simulink model "main_sim_mk14_final"  (R2024a)
settings: Solver=ode23t  StartTime=0.0  StopTime=0.2  MaxStep=5e-7  RelTol=1e-5
InitFcn:
  | sw_freq=40e3;
undefined symbols (not defined in the file or in its folder): Ion, Lithium
libraries: spsSeriesRLCBranchLib x10, spsMeanLib x8, spsCurrentMeasurementLib x6, spsMosfetLib x4, spsVoltageMeasurementLib x3, spsBatteryLib x2, simulink x2, spsControlledCurrentSourceLib x1, spsGroundLib x1, eeStairGenerator x1, spspowerguiLib x1
settings Model: SimulationMode=rapid-accelerator  Creator=adamo  LastModifiedBy=adamo
settings SolverCC: AllowMultiTaskInputOutput=on  ZeroCrossAlgorithm=Adaptive  SolverResetMethod=Robust  PositivePriorityOrder=on  DecoupledContinuousIntegration=on  MinimalZcImpactIntegration=on
settings OptimizationCC: ReuseModelBlockBuffer=off  SimCompilerOptimization=on
settings DebuggingCC: MaskedZcDiagnostic=none  IgnoredZcDiagnostic=none
settings HardwareCC: ProdHWDeviceType=AMD->x86-64 (Windows64)
settings ModelReferenceCC: EnableParallelModelReferenceBuilds=on  ParallelModelReferenceMATLABWorkerInit=Copy Base Workspace  ModelReferenceMinAlgLoopOccurrences=on
settings SFSimCC: SimHardwareAcceleration=native  SimTargetLang=C++
settings RTWCC: BuildConfiguration=Faster Runs  GPUComputeCapability=3.5
settings GRTTargetCC: OptimizeReductions=on

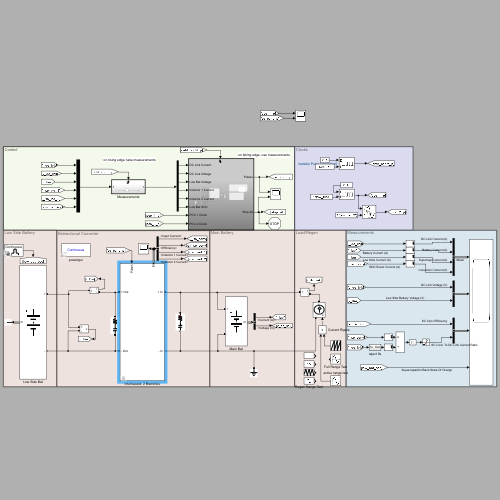
[thumbnail: Simulink's stored preview of the top-level diagram]
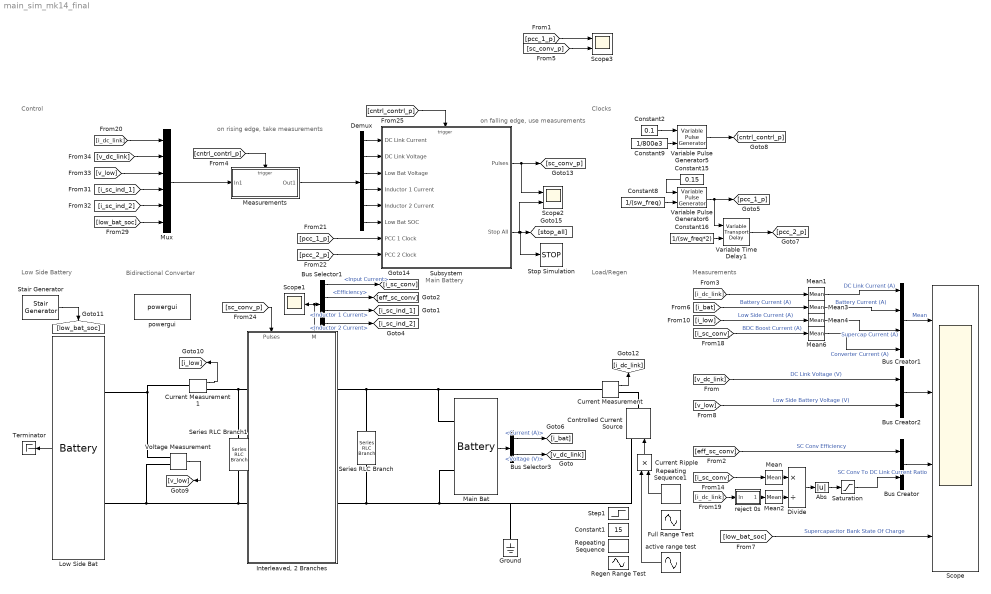
== system main_sim_mk14_final ==
  note: on falling edge, use measurements
  note: on rising edge, take measurements
  note: Clocks
  note: Control
  note: Measurements
  note: Bidirectional Converter
  note: Low Side Battery
  note: Main Battery
  note: Load/Regen
  Abs : Abs  SaturateOnIntegerOverflow=off
  Bus Creator : BusCreator  Inputs=2
  Bus Creator1 : BusCreator  Inputs=4
  Bus Creator2 : BusCreator  Inputs=2
  Bus Selector1 : BusSelector  OutputSignals=Input Current,Efficiency,Inductor 1 Current,Inductor 2 Current
  Bus Selector3 : BusSelector  OutputSignals=Current (A),Voltage (V)
  Constant1 : Constant  Value=15
  Constant15 : Constant  Value=0.15
  Constant16 : Constant  Value=1/(sw_freq*2)
  Constant2 : Constant  Value=0.1
  Constant8 : Constant  Value=1/(sw_freq)  VectorParams1D=off
  Constant9 : Constant  Value=1/800e3
  Controlled Current Source : spsControlledCurrentSourceLib/Controlled Current Source  Initialize=on  Source_Type=DC  Amplitude=0  Phase=0  Frequency=0  Measurements=None
  Current Measurement : spsCurrentMeasurementLib/Current Measurement  PhasorSimulation=off  OutputType=Complex  PSBequivalent=0
  Current Measurement1 : spsCurrentMeasurementLib/Current Measurement  PhasorSimulation=off  OutputType=Complex  PSBequivalent=0
  Current Ripple : Product
  Demux : Demux  Outputs=6
  Divide : Product  Inputs=*/
  Full Range Test : Sin  Amplitude=52  Frequency=314.1592/8  SampleTime=0
  Ground : spsGroundLib/Ground  LConnTagsString=a
  "Interleaved, 2 Branches" : Subsystem  mask{sw_freq_mean=sw_freq, ind_ind=200e-6, fet_res_on=10e-3, bd_d_for_volt=1.3}
      mask prompts: sw_freq_mean "Switching Frequency (Hz)"; ind_ind "Branch Inductor Inductance (H)"; fet_res_on "Drain-to-Source On-Resistance (Ohm)"; bd_d_for_volt "Body Diode Forward Voltage (V)"
      settings: PortSchema="{\"entries\":[{\"content\":{\"sides\":[{\"content\":{\"connectorIds\":[\"LConn1\",\"LConn2\"]},\"type\":\"ConnectorPlacement.EquallySpacedRectSide\",\"uuid\":\"57763a22-817d-4d04-a19a-6b084199baa7\"},{\"content\":{\"connectorIds\":[\"RConn1\",\"RConn2\"],\"side\":\"RIGHT\"},\"type\":\"ConnectorPlacement.EquallySpacedRectSide\",\"uuid\":\"e5f04f53-fac9-409a-ac58-f518a07f7aa1\"},{\"content\":{\"connectorIds\":[\"In1\",\"Out1\"],\"side\":\"TOP\"},\"type\":\"ConnectorPlacement.EquallySpacedRectSide\",\"uuid\":\"7683f119-33ed-4468-84c8-2aaaca937041\"}]},\"type\":\"ConnectorPlacement.EquallySpacedConnector\",\"uuid\":\"94c2a178-e796-4540-a87e-c79e0224e730\"}],\"packageUris\":[\"http://schema.mathworks.com/mf0/Connector/R2020b\"],\"version\":\"1.0\"}"
      mask DialogControl DescTextVar Prompt: %<MaskDescription>This block impements a Two Phase Interleaved Bidirectional DC-DC Buck/Boost Converter. Input is the left side (High Voltage Side). All MOSFETs share the same characteristics.
      mask DialogControl ParameterGroupVar Prompt: Circuit Parameters
      mask DialogControl Container3 Prompt: MOSFET Parameters
  Low Side Bat : spsBatteryLib/Battery  BatType=Lithium-Ion  ShowTempParam=off  ThermalPreset=no  ShowAgeParam=off  NomV=32  NomQ=30  SOC=75  Batt_Tr=30  PresetModel=on  MaxQ=30  MinV=24  FullV=37.2476  Dis_rate=13.0435  R=0.010667  Normal_OP=27.1304  expZone="[34.5723      1.47391]"  current=[6.5 13 32.5]  Units=Time  Tci=20  NomT=20  T2=-30  MaxQ2=4.8  FullV2=7.1  Normal_OP2=5.655  expZone2="[6.58           1]"  Rca=0.6  ti=2000  Dp=0  Neq0=0  Tsim=1e6  Ta1=25  Qeol=5.4*0.9  Reol=0.013333*1.2  Char_age=[2.3478, 3]  Dis_age=[2.3478, 10]  N1=1500  N2=10500  N3=1000  N4=1400  Ta2=45  N5=950
  Main Bat : spsBatteryLib/Battery  BatType=Lithium-Ion  ShowTempParam=off  ThermalPreset=no  ShowAgeParam=off  NomV=79  NomQ=100  SOC=75  Batt_Tr=30  PresetModel=on  MaxQ=100  MinV=59.25  FullV=91.955  Dis_rate=43.4783  R=0.0079  Normal_OP=90.4348  expZone="[85.3505      4.91304]"  current=[6.5 13 32.5]  Units=Time  Tci=20  NomT=20  T2=-30  MaxQ2=4.8  FullV2=7.1  Normal_OP2=5.655  expZone2="[6.58           1]"  Rca=0.6  ti=2000  Dp=0  Neq0=0  Tsim=1e6  Ta1=25  Qeol=5.4*0.9  Reol=0.013333*1.2  Char_age=[2.3478, 3]  Dis_age=[2.3478, 10]  N1=1500  N2=10500  N3=1000  N4=1400  Ta2=45  N5=950
  Mean : spsMeanLib/Mean  Freq=50e3/100  Vinit=0  Ts=0
  Mean{1,3..4,6} (4 alike) : spsMeanLib/Mean  Freq=50e3/10  Vinit=0  Ts=0
  Mean2 : spsMeanLib/Mean  Freq=50e3/100  Vinit=0  Ts=0
  Measurements : Subsystem  TreatAsAtomicUnit=on
  Mux : Mux  Inputs=6
  Regen Range Test : Sin  Amplitude=8  Bias=18  Frequency=314.1592/10  SampleTime=0
  Repeating Sequence : simulink/Sources/Repeating Sequence  rep_seq_t=[0 0.5 1]  rep_seq_y=[-20 60 -40]
  Repeating Sequence1 : simulink/Sources/Repeating Sequence  rep_seq_t=[0 0.0005]  rep_seq_y=[0.999 1]
  Saturation : Saturate  UpperLimit=1  LowerLimit=0
  Scope : Scope  NumInputPorts=4
  Scope1 : Scope
  Scope2 : Scope  NumInputPorts=2
  Scope3 : Scope  NumInputPorts=2
  Series RLC Branch : spsSeriesRLCBranchLib/Series RLC Branch  LConnTagsString=__new0  RConnTagsString=__new0  BranchType=RC  Resistance=1e-4  Inductance=1e-3  SetiL0=off  InitialCurrent=0  Capacitance=800e-6  Setx0=on  InitialVoltage=85  Measurements=None
  Series RLC Branch1 : spsSeriesRLCBranchLib/Series RLC Branch  LConnTagsString=__new0  RConnTagsString=__new0  BranchType=RC  Resistance=1e-4  Inductance=1e-3  SetiL0=off  InitialCurrent=0  Capacitance=400e-6  Setx0=on  InitialVoltage=35  Measurements=None
  Stair Generator : eeStairGenerator/Stair Generator  LabelModeActiveChoice=Continuous  TimeInput=[0 0.2 0.4 0.6 0.8]  AmplitudeInput=[30 50 95 50 30]  SampleTime=0  RepeatPattern=off  OutDataTypeStr=double
      settings: LibrarySourceBlock=ee_sl_lib/General Control/Stair Generator
  Step1 : Step  Time=0.1  Before=27  After=-25  SampleTime=0
  Stop Simulation : Stop
  Subsystem : Subsystem
  Terminator : Terminator
  Variable Time Delay1 : VariableTransportDelay  MaximumDelay=10  ZeroDelay=on
  Variable Pulse Generator5 : VariablePulseGenerator  AllowZeroPulseWidth=on  SampleTime=0.1
  Variable Pulse Generator6 : VariablePulseGenerator  AllowZeroPulseWidth=on  SampleTime=0.1
  Voltage Measurement : spsVoltageMeasurementLib/Voltage Measurement  PhasorSimulation=off  OutputType=Complex  PSBequivalent=0
  active range test : Sin  Amplitude=24  Bias=4  Frequency=314.1592/8  SampleTime=0
  powergui : spspowerguiLib/powergui  Priority=1  SimulationMode=Continuous  SampleTime=50e-6  frequency=60  Iterations=50  frequencyindice=0  Pbase=100e6  ErrMax=1e-4  UnitsV=kV  UnitsW=MW  buscounter=0  FunctionMessages=off  echomessages=off  EnableUseOfTLC=off  CurrentSourceSwitches=off  DisableSnubberDevices=on  DisableRonSwitches=off  DisableVfSwitches=off  DisplayEquations=off  AutomaticDiscreteSolvers=off  SolverType=Tustin/Backward Euler (TBE)  Interpol=off  ExternalGateDelay=off  methode=off  Ts=100  x0status=blocks  SPID=on  SwTol=0  HookPort=off  NonlinearTolerance=1e-4  nMaxIteration=100  ContinueOnMaxIteration=off  RestoreLinks=warning  ResistiveCurrentMeasurement=off  Frange=[0:2:500]  Ylog=off  Xlog=on  ShowGrid=off  save=off  variable=ZData  structure=0  ZoomFFT=off  StartTime=0.0  cycles=1  DisplayStyle=1  fundamental=60  FreqAxis=off  MaxFrequency=1000  frequencyindicesteady=1  RmsSteady=1  display=off
  reject 0s : Subsystem
  wires:
  [v_dc_link] -> Bus Creator2/1  "DC Link Voltage (V)"
  Bus Creator2/1 -> Scope/2
  Mean3/1 -> Bus Creator1/2  "Battery Current (A)"
  "Interleaved, 2 Branches"/1(M) -> Scope1/1, Bus Selector1/1
  [v_low] -> Bus Creator2/2  "Low Side Battery Voltage (V)"
  Mean4/1 -> Bus Creator1/3  "Supercap Current (A)"
  Bus Selector1/2 -> [eff_sc_conv]  "<Efficiency>"
  [eff_sc_conv] -> Bus Creator/1  "SC Conv Efficiency"
  [low_bat_soc] -> Scope/4  "Supercapacitor Bank State Of Charge"
  Bus Selector1/1 -> [i_sc_conv]  "<Input Current>"
  reject 0s/1(Out) -> Mean2/1
  Divide/1 -> Abs/1
  Abs/1 -> Saturation/1
  [i_sc_conv] -> Mean/1
  Saturation/1 -> Bus Creator/2  "SC Conv To DC Link Current Ratio"
  [i_dc_link] -> reject 0s/1(In)
  Bus Creator/1 -> Scope/3
  Bus Creator1/1 -> Scope/1  "Mean"
  Mean/1 -> Divide/1
  Mean2/1 -> Divide/2
  Mean1/1 -> Bus Creator1/1  "DC Link Current (A)"
  [i_bat] -> Mean3/1  "Battery Current (A)"
  [i_low] -> Mean4/1  "Low Side Current (A)"
  Mean6/1 -> Bus Creator1/4  "Converter Current (A)"
  [i_sc_conv] -> Mean6/1  "BDC Boost Current (A)"
  [sc_conv_p] -> "Interleaved, 2 Branches"/1(Pulses)
  Bus Selector3/2 -> [v_dc_link]  "<Voltage (V)>"
  Bus Selector3/1 -> [i_bat]  "<Current (A)>"
  [i_dc_link] -> Mean1/1
  Current Measurement/1 -> [i_dc_link]
  Main Bat/1 -> Bus Selector3/1
  Bus Selector1/3 -> [i_sc_ind_1]  "<Inductor 1 Current>"
  Bus Selector1/4 -> [i_sc_ind_2]  "<Inductor 2 Current>"
  Voltage Measurement/1 -> [v_low]
  Current Measurement1/1 -> [i_low]
  Repeating Sequence1/1 -> Current Ripple/2
  Current Ripple/1 -> Controlled Current Source/1
  Constant16/1 -> Variable Time Delay1/2
  Constant8/1 -> Variable Pulse Generator6/2
  Constant15/1 -> Variable Pulse Generator6/1
  Variable Pulse Generator6/1 -> Variable Time Delay1/1, [pcc_1_p]
  Variable Time Delay1/1 -> [pcc_2_p]
  Constant2/1 -> Variable Pulse Generator5/1
  Constant9/1 -> Variable Pulse Generator5/2
  Variable Pulse Generator5/1 -> [cntrl_contrl_p]
  [cntrl_contrl_p] -> Subsystem/Trigger
  Subsystem/1(Pulses) -> Scope2/1, [sc_conv_p]
  active range test/1 -> Current Ripple/1
  [low_bat_soc] -> Mux/6
  [i_sc_ind_2] -> Mux/5
  [i_sc_ind_1] -> Mux/4
  [v_low] -> Mux/3
  [v_dc_link] -> Mux/2
  [i_dc_link] -> Mux/1
  Demux/1 -> Subsystem/1(DC Link Current)
  Demux/2 -> Subsystem/2(DC Link Voltage)
  Demux/3 -> Subsystem/3(Low Bat Voltage)
  Demux/5 -> Subsystem/5(Inductor 2 Current)
  Demux/4 -> Subsystem/4(Inductor 1 Current)
  Demux/6 -> Subsystem/6(Low Bat SOC)
  Measurements/1(Out1) -> Demux/1
  Mux/1 -> Measurements/1(In1)
  [cntrl_contrl_p] -> Measurements/Trigger
  Low Side Bat/1 -> Terminator/1
  Stair Generator/1 -> [low_bat_soc]
  Subsystem/2(Stop All) -> Scope2/2, Stop Simulation/1, [stop_all]
  [pcc_1_p] -> Scope3/1
  [sc_conv_p] -> Scope3/2
  [pcc_1_p] -> Subsystem/7(PCC 1 Clock)
  [pcc_2_p] -> Subsystem/8(PCC 2 Clock)
  connections:
  Series RLC Branch/RConn1 -- Controlled Current Source/LConn1 -- Ground/LConn1 -- Main Bat/LConn2 -- "Interleaved, 2 Branches"/RConn2
  "Interleaved, 2 Branches"/LConn2 -- Series RLC Branch1/RConn1 -- Low Side Bat/LConn2 -- Voltage Measurement/LConn2
  Controlled Current Source/RConn1 -- Current Measurement/RConn1
  Voltage Measurement/LConn1 -- Low Side Bat/LConn1 -- Current Measurement1/LConn1
  Current Measurement/LConn1 -- "Interleaved, 2 Branches"/RConn1 -- Series RLC Branch/LConn1 -- Main Bat/LConn1
  "Interleaved, 2 Branches"/LConn1 -- Series RLC Branch1/LConn1 -- Current Measurement1/RConn1

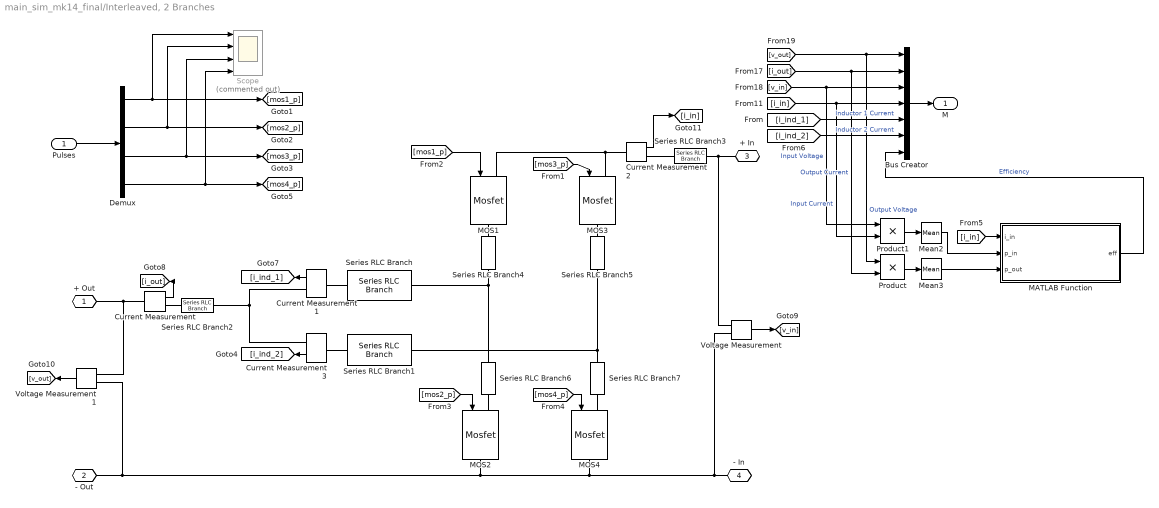
== system main_sim_mk14_final/Interleaved, 2 Branches ==
  Pulses : Inport
  Bus Creator : BusCreator  Inputs=7
  Current Measurement{,1..3} (4 alike) : spsCurrentMeasurementLib/Current Measurement  PhasorSimulation=off  OutputType=Complex  PSBequivalent=0
  Demux : Demux
  MATLAB Function : MATLAB Function  TreatAsAtomicUnit=on
  MOS{1..4} (4 alike) : spsMosfetLib/Mosfet  Ron=fet_res_on  Lon=0  Rd=0.01  Vfd=bd_d_for_volt  IC=0  Rs=1e5  Cs=inf  Measurements=off
  Mean2 : spsMeanLib/Mean  Freq=sw_freq_mean/10  Vinit=0  Ts=0
  Mean3 : spsMeanLib/Mean  Freq=sw_freq_mean/10  Vinit=0  Ts=0
  Product : Product
  Product1 : Product
  Scope : Scope  Commented=on  NumInputPorts=4
  Series RLC Branch : spsSeriesRLCBranchLib/Series RLC Branch  LConnTagsString=__new0  RConnTagsString=__new0  BranchType=RL  Resistance=1e-3  Inductance=ind_ind  SetiL0=off  InitialCurrent=1e-3  Capacitance=1e-6  Setx0=off  InitialVoltage=0  Measurements=None
  Series RLC Branch1 : spsSeriesRLCBranchLib/Series RLC Branch  LConnTagsString=__new0  RConnTagsString=__new0  BranchType=RL  Resistance=1e-3  Inductance=ind_ind  SetiL0=off  InitialCurrent=1e-3  Capacitance=1e-6  Setx0=off  InitialVoltage=0  Measurements=None
  Series RLC Branch2 : spsSeriesRLCBranchLib/Series RLC Branch  LConnTagsString=__new0  RConnTagsString=__new0  BranchType=R  Resistance=10e-3  Inductance=5e-4  SetiL0=off  InitialCurrent=1e-3  Capacitance=1e-6  Setx0=off  InitialVoltage=0  Measurements=None
  Series RLC Branch3 : spsSeriesRLCBranchLib/Series RLC Branch  LConnTagsString=__new0  RConnTagsString=__new0  BranchType=R  Resistance=10e-3  Inductance=5e-4  SetiL0=off  InitialCurrent=1e-3  Capacitance=1e-6  Setx0=off  InitialVoltage=0  Measurements=None
  Series RLC Branch{4..7} (4 alike) : spsSeriesRLCBranchLib/Series RLC Branch  LConnTagsString=__new0  RConnTagsString=__new0  BranchType=R  Resistance=1e-3  Inductance=5e-4  SetiL0=off  InitialCurrent=1e-3  Capacitance=1e-6  Setx0=off  InitialVoltage=0  Measurements=None
  Voltage Measurement : spsVoltageMeasurementLib/Voltage Measurement  PhasorSimulation=off  OutputType=Complex  PSBequivalent=0
  Voltage Measurement1 : spsVoltageMeasurementLib/Voltage Measurement  PhasorSimulation=off  OutputType=Complex  PSBequivalent=0
  + Out : PMIOPort  Side=Left
  - Out : PMIOPort  Port=2  Side=Left
  "+ In " : PMIOPort  Port=3  Side=Right
  "- In " : PMIOPort  Port=4  Side=Right
  M : Outport
  wires:
  [mos1_p] -> MOS1/1
  [mos2_p] -> MOS2/1
  Current Measurement1/1 -> [i_ind_1]
  Current Measurement2/1 -> [i_in]
  Voltage Measurement1/1 -> [v_out]
  Voltage Measurement/1 -> [v_in]
  [i_ind_2] -> Bus Creator/6  "Inductor 2 Current"
  Bus Creator/1 -> M/1
  [v_in] -> Bus Creator/3, Product1/1  "Input Voltage"
  [i_out] -> Product/2, Bus Creator/2  "Output Current"
  [i_in] -> Product1/2, Bus Creator/4  "Input Current"
  [v_out] -> Product/1, Bus Creator/1  "Output Voltage"
  MATLAB Function/1(eff) -> Bus Creator/7  "Efficiency"
  Product/1 -> Mean3/1
  Product1/1 -> Mean2/1
  [i_in] -> MATLAB Function/1(i_in)
  Pulses/1 -> Demux/1
  Demux/1 -> Scope/1, [mos1_p]
  Mean2/1 -> MATLAB Function/2(p_in)
  Mean3/1 -> MATLAB Function/3(p_out)
  Current Measurement/1 -> [i_out]
  [mos3_p] -> MOS3/1
  Current Measurement3/1 -> [i_ind_2]
  [i_ind_1] -> Bus Creator/5  "Inductor 1 Current"
  Demux/3 -> Scope/3, [mos3_p]
  Demux/4 -> Scope/4, [mos4_p]
  Demux/2 -> Scope/2, [mos2_p]
  [mos4_p] -> MOS4/1
  connections:
  MOS1/LConn1 -- Current Measurement2/LConn1 -- MOS3/LConn1
  Voltage Measurement1/LConn1 -- Current Measurement/LConn1 -- + Out/RConn1
  "+ In "/RConn1 -- Voltage Measurement/LConn1 -- Series RLC Branch3/RConn1
  "- In "/RConn1 -- Voltage Measurement/LConn2 -- Voltage Measurement1/LConn2 -- - Out/RConn1 -- MOS2/RConn1 -- MOS4/RConn1
  Series RLC Branch/LConn1 -- Current Measurement1/LConn1
  Series RLC Branch/RConn1 -- Series RLC Branch6/LConn1 -- Series RLC Branch4/RConn1
  Series RLC Branch1/RConn1 -- Series RLC Branch7/LConn1 -- Series RLC Branch5/RConn1
  Series RLC Branch1/LConn1 -- Current Measurement3/LConn1
  Series RLC Branch2/RConn1 -- Current Measurement3/RConn1 -- Current Measurement1/RConn1
  Series RLC Branch2/LConn1 -- Current Measurement/RConn1
  Series RLC Branch4/LConn1 -- MOS1/RConn1
  Series RLC Branch5/LConn1 -- MOS3/RConn1
  Series RLC Branch6/RConn1 -- MOS2/LConn1
  Series RLC Branch7/RConn1 -- MOS4/LConn1
  Series RLC Branch3/LConn1 -- Current Measurement2/RConn1

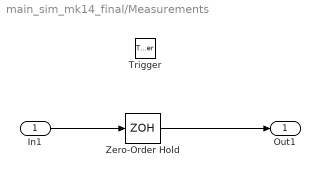
== system main_sim_mk14_final/Measurements ==
  In1 : Inport
  Trigger : TriggerPort  VariantControl=(inherit)
  Zero-Order Hold : ZeroOrderHold  SampleTime=-1
  Out1 : Outport
  wires:
  In1/1 -> Zero-Order Hold/1
  Zero-Order Hold/1 -> Out1/1

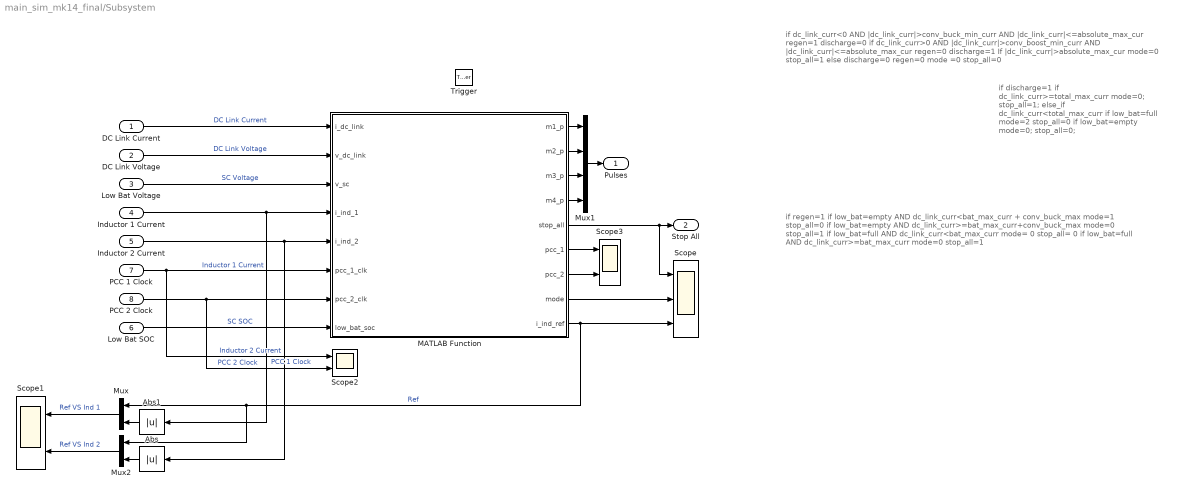
== system main_sim_mk14_final/Subsystem ==
  note: if regen=1
      | 	if low_bat=empty AND dc_link_curr<bat_max_curr + conv_buck_max
      | 		mode=1
      | 		stop_all=0
      | 	if low_bat=empty AND dc_link_curr>=bat_max_curr+conv_buck_max
      | 		mode=0
      | 		stop_all=1
      | 	if low_bat=full AND dc_link_curr<bat_max_curr
      | 		mode= 0
      | 		stop_all= 0
      | 	if low_bat=full AND dc_link_curr>=bat_max_curr
      | 		mode=0
      | 		stop_all=1
  note: if discharge=1
      | 	if dc_link_curr>=total_max_curr
      | 		mode=0;
      | 		stop_all=1;
      | 	else_if dc_link_curr<total_max_curr
      | 		if low_bat=full
      | 			mode=2
      | 			stop_all=0
      | 		if low_bat=empty
      | 			mode=0;
      | 			stop_all=0;
  note: if dc_link_curr<0 AND |dc_link_curr|>conv_buck_min_curr AND |dc_link_curr|<=absolute_max_cur
      | 	regen=1
      | 	discharge=0
      | if dc_link_curr>0 AND |dc_link_curr|>conv_boost_min_curr AND |dc_link_curr|<=absolute_max_cur
      | 	regen=0
      | 	discharge=1
      | If  |dc_link_curr|>absolute_max_cur
      | 	mode=0
      | 	stop_all=1
      | else
      | 	discharge=0
      | 	regen=0
      | 	mode =0
      | 	stop_all=0
  DC Link Current : Inport
  DC Link Voltage : Inport  Port=2
  Low Bat Voltage : Inport  Port=3
  Inductor 1 Current : Inport  Port=4
  Inductor 2 Current : Inport  Port=5
  Low Bat SOC : Inport  Port=6
  PCC 1 Clock : Inport  Port=7
  PCC 2 Clock : Inport  Port=8
  Trigger : TriggerPort  TriggerType=falling  VariantControl=(inherit)  PortDimensions=1
  Abs : Abs  SaturateOnIntegerOverflow=off
  Abs1 : Abs  SaturateOnIntegerOverflow=off
  MATLAB Function : MATLAB Function  TreatAsAtomicUnit=on
  Mux : Mux  Inputs=2
  Mux1 : Mux
  Mux2 : Mux  Inputs=2
  Scope : Scope  NumInputPorts=3
  Scope1 : Scope  NumInputPorts=2
  Scope2 : Scope  NumInputPorts=2
  Scope3 : Scope  NumInputPorts=2
  Pulses : Outport
  Stop All : Outport  Port=2
  wires:
  MATLAB Function/1(m1_p) -> Mux1/1
  PCC 2 Clock/1 -> MATLAB Function/7(pcc_2_clk), Scope2/2  "PCC 2 Clock"
  DC Link Voltage/1 -> MATLAB Function/2(v_dc_link)  "DC Link Voltage"
  MATLAB Function/2(m2_p) -> Mux1/2
  Mux1/1 -> Pulses/1
  DC Link Current/1 -> MATLAB Function/1(i_dc_link)  "DC Link Current"
  Low Bat Voltage/1 -> MATLAB Function/3(v_sc)  "SC Voltage"
  Inductor 1 Current/1 -> MATLAB Function/4(i_ind_1), Abs1/1  "Inductor 1 Current"
  Low Bat SOC/1 -> MATLAB Function/8(low_bat_soc)  "SC SOC"
  MATLAB Function/5(stop_all) -> Scope/1, Stop All/1
  Inductor 2 Current/1 -> MATLAB Function/5(i_ind_2), Abs/1  "Inductor 2 Current"
  PCC 1 Clock/1 -> Scope2/1, MATLAB Function/6(pcc_1_clk)  "PCC 1 Clock"
  MATLAB Function/8(mode) -> Scope/2
  MATLAB Function/9(i_ind_ref) -> Mux/1, Mux2/1, Scope/3  "Ref"
  Mux/1 -> Scope1/1  "Ref VS Ind 1"
  Mux2/1 -> Scope1/2  "Ref VS Ind 2"
  Abs/1 -> Mux2/2
  Abs1/1 -> Mux/2
  MATLAB Function/6(pcc_1) -> Scope3/1
  MATLAB Function/7(pcc_2) -> Scope3/2
  MATLAB Function/3(m3_p) -> Mux1/3
  MATLAB Function/4(m4_p) -> Mux1/4

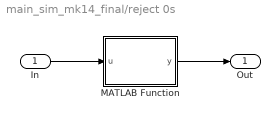
== system main_sim_mk14_final/reject 0s ==
  In : Inport
  MATLAB Function : MATLAB Function  TreatAsAtomicUnit=on
  Out : Outport
  wires:
  MATLAB Function/1(y) -> Out/1
  In/1 -> MATLAB Function/1(u)

== matlab function main_sim_mk14_final/Subsystem/MATLAB Function ==
  data: i_dc_link input; m1_p output; v_dc_link input; v_sc input; i_ind_1 input; i_ind_2 input; pcc_1_clk input; pcc_2_clk input; low_bat_soc input; m2_p output; m3_p output; m4_p output; stop_all output; pcc_1 output; pcc_2 output; mode output; i_ind_ref output
function [m1_p,m2_p,m3_p,m4_p,stop_all,pcc_1,pcc_2,mode,i_ind_ref]= call_central_cntrl(i_dc_link,v_dc_link,v_sc,i_ind_1,i_ind_2,pcc_1_clk,pcc_2_clk,low_bat_soc)


[m1_p,m2_p,m3_p,m4_p,stop_all,pcc_1,pcc_2,mode,i_ind_ref]=central_cntrl(i_dc_link,v_dc_link,v_sc,i_ind_1,i_ind_2,pcc_1_clk,pcc_2_clk,low_bat_soc);

== matlab function main_sim_mk14_final/reject 0s/MATLAB Function ==
  data: u input; y output
function y = fcn(u)
if u==0
    y=0.001;
else 
    y=u;
end
y = u;

== matlab function main_sim_mk14_final/Interleaved, 2 Branches/MATLAB Function ==
  data: i_in input; eff output; p_in input; p_out input
function eff = eff_calc(i_in,p_in,p_out)

if i_in>=0
    eff=min(max(p_in/p_out,0),1);
else
    eff=min(max(p_out/p_in,0),1);
end
